simulink model "CircuitInterface"  (R2023b)
settings: configuration reference "Configuration" (kept outside this file)
undefined symbols (not defined in the file): SWITCH_STATE_e
settings Model: Creator=leona  LastModifiedBy=leona
settings ConfigSetRef: SourceName=Configuration  SourceLocation=Base Workspace

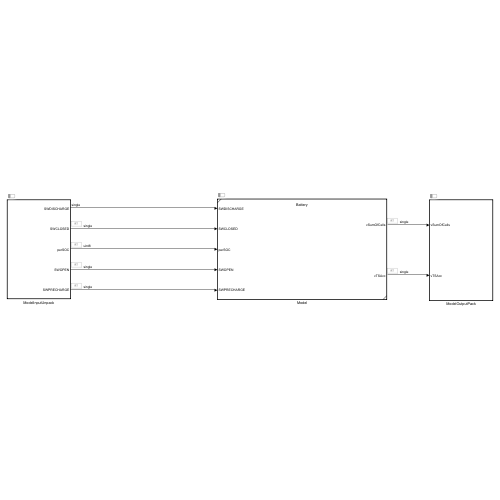
[thumbnail: Simulink's stored preview of the top-level diagram]
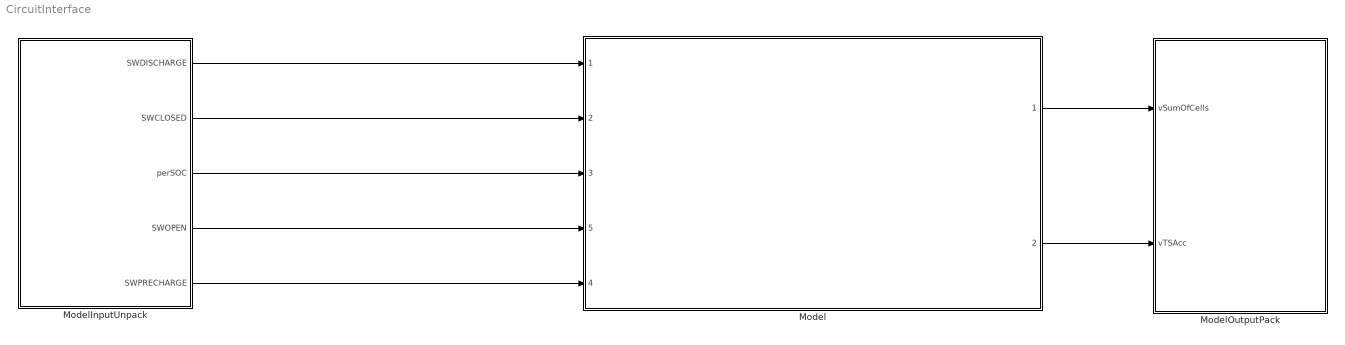
== system CircuitInterface ==
  Model : Subsystem  TreatAsAtomicUnit=on  ScheduleAs=Periodic partition  PartitionName=CiruitSubsystem  SystemSampleTime=0.005  ReferencedSubsystem=Battery
      settings: PortSchema="{\"entries\":[{\"content\":{\"sides\":[{\"content\":{\"connectorIds\":[\"In1\",\"In2\",\"In3\",\"In5\",\"In4\"]},\"type\":\"ConnectorPlacement.EquallySpacedRectSide\",\"uuid\":\"5e4423b7-0677-4123-82e8-52544a0245db\"},{\"content\":{\"connectorIds\":[\"Out1\",\"Out2\"],\"side\":\"RIGHT\"},\"type\":\"ConnectorPlacement.EquallySpacedRectSide\",\"uuid\":\"94cda0c5-634b-427a-a30c-cf0e3dec8d4f\"},{\"content\":{\"side\":\"TOP\"},\"type\":\"ConnectorPlacement.EquallySpacedRectSide\",\"uuid\":\"49c1d658-8010-4cbb-a2d4-2d9f82befc76\"}]},\"type\":\"ConnectorPlacement.EquallySpacedConnector\",\"uuid\":\"dc3a2f53-99fc-4e14-ada0-996178b95a62\"}],\"packageUris\":[\"http://schema.mathworks.com/mf0/Connector/R2020b\"],\"version\":\"1.0\"}"
  ModelInputUnpack : Subsystem  Priority=1  TreatAsAtomicUnit=on  ScheduleAs=Periodic partition  PartitionName=ModelInputUnpack  SystemSampleTime=0.005
  ModelOutputPack : Subsystem  Priority=3  TreatAsAtomicUnit=on  ScheduleAs=Periodic partition  PartitionName=ModelOutputPack  SystemSampleTime=0.005
  wires:
  ModelInputUnpack/2(SWCLOSED) -> Model/2
  ModelInputUnpack/3(perSOC) -> Model/3
  Model/1 -> ModelOutputPack/1(vSumOfCells)
  Model/2 -> ModelOutputPack/2(vTSAcc)
  ModelInputUnpack/1(SWDISCHARGE) -> Model/1
  ModelInputUnpack/4(SWOPEN) -> Model/5
  ModelInputUnpack/5(SWPRECHARGE) -> Model/4

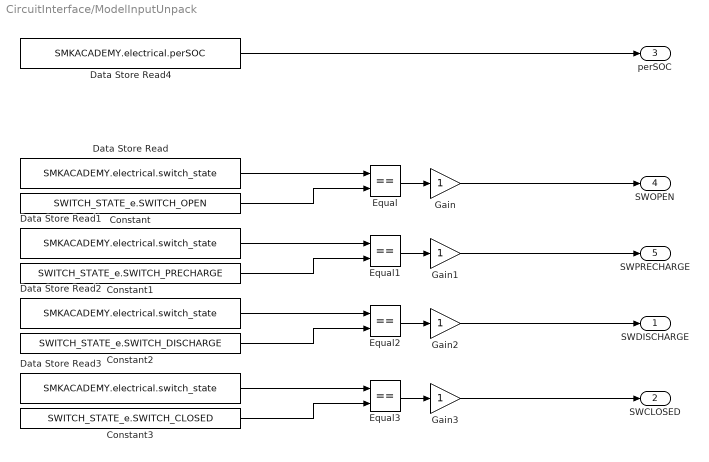
== system CircuitInterface/ModelInputUnpack ==
  Constant : Constant  Value=SWITCH_STATE_e.SWITCH_OPEN
  Constant1 : Constant  Value=SWITCH_STATE_e.SWITCH_PRECHARGE
  Constant2 : Constant  Value=SWITCH_STATE_e.SWITCH_DISCHARGE
  Constant3 : Constant  Value=SWITCH_STATE_e.SWITCH_CLOSED
  Data Store Read{,1..3} (4 alike) : DataStoreRead  DataStoreName=SMKACADEMY  DataStoreElements=SMKACADEMY.electrical.switch_state  IndexOptions=Index vector (dialog)  Indices=1  OutputSizes=1
  Data Store Read4 : DataStoreRead  DataStoreName=SMKACADEMY  DataStoreElements=SMKACADEMY.electrical.perSOC  IndexOptions=Index vector (dialog)  Indices=1  OutputSizes=1
  Equal{,1..3} (4 alike) : RelationalOperator  Operator===  OutDataTypeStr=boolean  RndMeth=Simplest  InputSameDT=off
  Gain{,1..3} (4 alike) : Gain  OutDataTypeStr=single
  SWDISCHARGE : Outport
  SWCLOSED : Outport  Port=2
  perSOC : Outport  Port=3
  SWOPEN : Outport  Port=4
  SWPRECHARGE : Outport  Port=5
  wires:
  Equal/1 -> Gain/1
  Gain/1 -> SWOPEN/1
  Constant/1 -> Equal/2
  Data Store Read/1 -> Equal/1
  Data Store Read1/1 -> Equal1/1
  Equal1/1 -> Gain1/1
  Constant1/1 -> Equal1/2
  Data Store Read2/1 -> Equal2/1
  Equal2/1 -> Gain2/1
  Constant2/1 -> Equal2/2
  Data Store Read3/1 -> Equal3/1
  Equal3/1 -> Gain3/1
  Constant3/1 -> Equal3/2
  Gain1/1 -> SWPRECHARGE/1
  Gain2/1 -> SWDISCHARGE/1
  Gain3/1 -> SWCLOSED/1
  Data Store Read4/1 -> perSOC/1

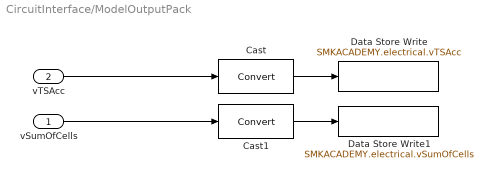
== system CircuitInterface/ModelOutputPack ==
  vSumOfCells : Inport
  vTSAcc : Inport  Port=2
  Cast : DataTypeConversion  SaturateOnIntegerOverflow=off  RndMeth=Floor
  Cast1 : DataTypeConversion  SaturateOnIntegerOverflow=off  RndMeth=Floor
  Data Store Write : DataStoreWrite  DataStoreName=SMKACADEMY  DataStoreElements=SMKACADEMY.electrical.vTSAcc  IndexOptions=Index vector (dialog)  Indices=1  OutputSizes=1
  Data Store Write1 : DataStoreWrite  DataStoreName=SMKACADEMY  DataStoreElements=SMKACADEMY.electrical.vSumOfCells  IndexOptions=Index vector (dialog)  Indices=1  OutputSizes=1
  wires:
  vTSAcc/1 -> Cast/1
  Cast/1 -> Data Store Write/1
  vSumOfCells/1 -> Cast1/1
  Cast1/1 -> Data Store Write1/1
